simulink model "SF014A_InertiaCmpVel"  (R2013b)
settings: Solver=FixedStepDiscrete  SolverMode=SingleTasking  StartTime=0.0  StopTime=10  FixedStep=0.002  RelTol=1e-3
undefined symbols (not defined in the file): ARCHGLBPRM_2MILLISEC_SEC_F32, ARCHGLBPRM_2PI_ULS_F32, ARCHGLBPRM_PIOVER180_ULS_F32, FLTINJ_INERTIACMPVEL_INERTIACMPCMD, InertiaCmpVelDampgDecelGain, InertiaCmpVelDampgDecelGainFallSlew, InertiaCmpVelDampgGainOffThd, InertiaCmpVelDampgGainOnThd, InertiaCmpVelDecelGainEnaCal, InertiaCmpVelMotInertia, InertiaCmpVelNotchFilStruct, NOTCHFILZEROTHD_ULS_F32, SysGlbPrmSysKineRat, SysGlbPrmTorsBarStfn
libraries: FixdToFloat x13, LnrIntrpn x13, FloatToFixd x9, NxtrAbslt x4, NxtrMath x4, NxtrLim x4, simulink x2, Fil x2
(part 2 of 3)

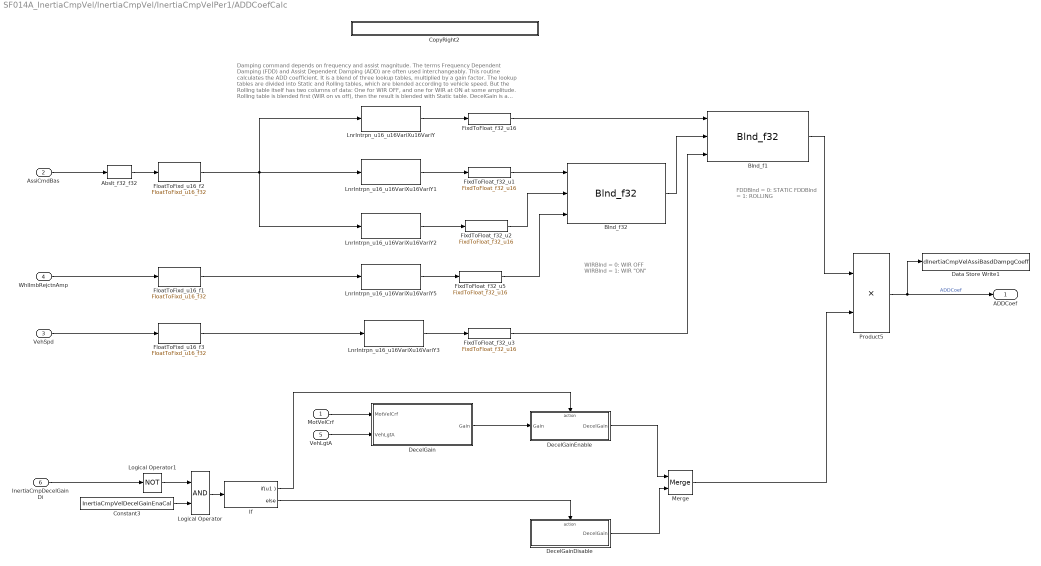
== system SF014A_InertiaCmpVel/InertiaCmpVel/InertiaCmpVelPer1/ADDCoefCalc ==
  note: Damping command depends on frequency and assist magnitude.  The terms Frequency Dependent Damping (FDD) and Assist Dependent Damping (ADD) are
      | often used interchangeably.  This routine calculates the ADD coefficient.  It is a blend of three lookup tables, multiplied by a gain factor.  The lookup tables
      | are divided into Static and Rolling tables, which are blended according to vehicle speed.  But the Rolling table itself has two columns of data:  One for
      | WIR OFF, and one for WIR at ON at some amplitude.  Rolling table is blended first (WIR on vs off), then the result is blended with Static table.
      |
      | DecelGain is a gain applied to damping coefficient when vehicle is aggressively decelerating.
  note: FDDBlnd = 0:  STATIC
      | FDDBlnd = 1:  ROLLING
  note: WIRBlnd = 0:  WIR OFF
      | WIRBlnd = 1:  WIR "ON"
  MotVelCrf : Inport  RequirementInfo="{'linktype_rmi_doors' '0000a52e (/E-STEER Core/SubSystem Specifications/Application Functions/SF014A Inertia Compensation)' '#SF014A_76' 'true' 'REQ:  SF014A_76' '' } %GIDa_dfa7856d_1c61_4589_b30e_750f1eb1645f"
  AssiCmdBas : Inport  RequirementInfo="{'linktype_rmi_doors' '0000a52e (/E-STEER Core/SubSystem Specifications/Application Functions/SF014A Inertia Compensation)' '#SF014A_78' 'true' 'REQ:  SF014A_78' '' } %GIDa_f4af5cbb_f21a_47bc_a42f_a4172f088ae5"  Port=2
  VehSpd : Inport  RequirementInfo="{'linktype_rmi_doors' '0000a52e (/E-STEER Core/SubSystem Specifications/Application Functions/SF014A Inertia Compensation)' '#SF014A_79' 'true' 'REQ:  SF014A_79' '' } %GIDa_a01f0a88_c757_4666_8b69_1ba2342a6170"  Port=3
  WhlImbRejctnAmp : Inport  RequirementInfo="{'linktype_rmi_doors' '0000a52e (/E-STEER Core/SubSystem Specifications/Application Functions/SF014A Inertia Compensation)' '#SF014A_75' 'true' 'REQ:  SF014A_75' '' } %GIDa_85975baa_77aa_432b_910d_ccf6f040e7b8"  Port=4
  VehLgtA : Inport  RequirementInfo="{'linktype_rmi_doors' '0000a52e (/E-STEER Core/SubSystem Specifications/Application Functions/SF014A Inertia Compensation)' '#SF014A_76' 'true' 'REQ:  SF014A_76' '' } %GIDa_8e8fb2ce_6071_474e_9d78_82a4e9de4257"  Port=5
  InertiaCmpDecelGainDi : Inport  RequirementInfo="{'linktype_rmi_doors' '0000a52e (/E-STEER Core/SubSystem Specifications/Application Functions/SF014A Inertia Compensation)' '#SF014A_80' 'true' 'REQ:  SF014A_80' '' } %GIDa_37223524_d1af_4ae4_9408_3e29b9ebc95d"  Port=6
  Abslt_f32_f32 : NxtrAbslt/Abslt_f32_f32  RequirementInfo="{'linktype_rmi_doors' '0000a52e (/E-STEER Core/SubSystem Specifications/Application Functions/SF014A Inertia Compensation)' '#SF014A_78' 'true' 'REQ:  SF014A_78' '' } %GIDa_af49941a_3ea7_4a2b_9c86_73a97f0de25e"  SFunctionSpec=single y1 = Abslt_f32_f32(single u1)
      settings: AttributesFormatString=%<Name>
  Blnd_f1 : NxtrMath/Blnd_f32  RequirementInfo="{'linktype_rmi_doors' '0000a52e (/E-STEER Core/SubSystem Specifications/Application Functions/SF014A Inertia Compensation)' '#SF014A_77' 'true' 'REQ:  SF014A_77' '' } %GIDa_d5de407a_03b4_47a0_a0b7_c554db3a096e"  SFunctionSpec=single y1 = Blnd_f32(single u1, single u2, single u3)  Parameter3=on
      settings: AttributesFormatString=%<Name>
  Blnd_f32 : NxtrMath/Blnd_f32  RequirementInfo="{'linktype_rmi_doors' '0000a52e (/E-STEER Core/SubSystem Specifications/Application Functions/SF014A Inertia Compensation)' '#SF014A_78' 'true' 'REQ:  SF014A_78' '' } %GIDa_356698f6_9f19_4ce5_b1f0_7f4a0c72e2f1"  SFunctionSpec=single y1 = Blnd_f32(single u1, single u2, single u3)  Parameter3=on
      settings: AttributesFormatString=%<Name>
  Constant3 : Constant  RequirementInfo="{'linktype_rmi_doors' '0000a52e (/E-STEER Core/SubSystem Specifications/Application Functions/SF014A Inertia Compensation)' '#SF014A_80' 'true' 'REQ:  SF014A_80' '' } %GIDa_3db1bff2_4e73_4e4e_8f98_1cb123555da8"  Value=InertiaCmpVelDecelGainEnaCal  OutDataTypeStr=boolean
  CopyRight2 : Subsystem  Description=|  mask(Copyright Information){none=on}
      | Copyright info block.                                               
      |                                                                     
      | Place copyright information at the top of every subsystem in design.
      mask prompts: none "No parameters"
      mask help: Place copyright information at the top of every subsystem in design.
      mask Display:
      | NxtrConf = 'Nexteer Confidential';
      | 
      | sys = bdroot; %handle for the current model ("system")
      | first = get_param(sys,'Created');
      | first = first(end-3:end);  %year is last four digits
      | 
      | last = get_param(sys,'LastModifiedDate');
      | if isempty(last)
      |     last = datestr(now,'yyyy');
      | else
      |     last = last(end-3:end);
      | end
      | 
      | if strcmp(first,last)
      |     fprintf('%s -- Copyright %s Nexteer',NxtrConf,first)
      | else
      |     fprintf('%s -- %s%s- %s Nexteer',NxtrConf,char(169),first,last)
      | end
  Data Store Write1 : DataStoreWrite  RequirementInfo="{'linktype_rmi_doors' '0000a52e (/E-STEER Core/SubSystem Specifications/Application Functions/SF014A Inertia Compensation)' '#SF014A_60' 'true' 'REQ:  SF014A_60' '' } %GIDa_70e6b0ec_6545_4ee6_978e_0c2c9530ad6e"  DataStoreName=dInertiaCmpVelAssiBasdDampgCoeff
  DecelGain : Subsystem  RequirementInfo="{'linktype_rmi_doors' '0000a52e (/E-STEER Core/SubSystem Specifications/Application Functions/SF014A Inertia Compensation)' '#SF014A_76' 'true' 'REQ:  SF014A_76' '' } %GIDa_fe0741f4_7d15_4f25_a644_7e9186648f35"
  DecelGainDisable : Subsystem  RequirementInfo="{'linktype_rmi_doors' '0000a52e (/E-STEER Core/SubSystem Specifications/Application Functions/SF014A Inertia Compensation)' '#SF014A_80' 'true' 'REQ:  SF014A_80' '' } %GIDa_c6f53ddd_25da_4339_8f12_9028726cb779"  TreatAsAtomicUnit=on
  DecelGainEnable : Subsystem  RequirementInfo="{'linktype_rmi_doors' '0000a52e (/E-STEER Core/SubSystem Specifications/Application Functions/SF014A Inertia Compensation)' '#SF014A_76' 'true' 'REQ:  SF014A_76' '' } %GIDa_e8d06ef6_defe_46f5_9046_6e95b5ce97d1"  TreatAsAtomicUnit=on
  FixdToFloat_f32_u1 : FixdToFloat/FixdToFloat_f32_u16  RequirementInfo="{'linktype_rmi_doors' '0000a52e (/E-STEER Core/SubSystem Specifications/Application Functions/SF014A Inertia Compensation)' '#SF014A_78' 'true' 'REQ:  SF014A_78' '' } %GIDa_be224bf3_1cd8_491e_b2d0_ce3df0214372"  Param1=16
  FixdToFloat_f32_u16 : FixdToFloat/FixdToFloat_f32_u16  RequirementInfo="{'linktype_rmi_doors' '0000a52e (/E-STEER Core/SubSystem Specifications/Application Functions/SF014A Inertia Compensation)' '#SF014A_77' 'true' 'REQ:  SF014A_77' '' } %GIDa_c4e94e59_b1c9_4f1f_9b7c_e38f7fa17322"  Param1=16
  FixdToFloat_f32_u2 : FixdToFloat/FixdToFloat_f32_u16  RequirementInfo="{'linktype_rmi_doors' '0000a52e (/E-STEER Core/SubSystem Specifications/Application Functions/SF014A Inertia Compensation)' '#SF014A_78' 'true' 'REQ:  SF014A_78' '' } %GIDa_4a949351_78f0_49de_9203_28cc4f0a5888"  Param1=16
  FixdToFloat_f32_u3 : FixdToFloat/FixdToFloat_f32_u16  RequirementInfo="{'linktype_rmi_doors' '0000a52e (/E-STEER Core/SubSystem Specifications/Application Functions/SF014A Inertia Compensation)' '#SF014A_79' 'true' 'REQ:  SF014A_79' '' } %GIDa_c7f288c6_8432_4513_b88a_c2722fb22052"  Param1=15
  FixdToFloat_f32_u5 : FixdToFloat/FixdToFloat_f32_u16  RequirementInfo="{'linktype_rmi_doors' '0000a52e (/E-STEER Core/SubSystem Specifications/Application Functions/SF014A Inertia Compensation)' '#SF014A_75' 'true' 'REQ:  SF014A_75' '' } %GIDa_6d830592_a8f2_4eeb_a9c7_97a648ca295c"  Param1=15
  FloatToFixd_u16_f1 : FloatToFixd/FloatToFixd_u16_f32  RequirementInfo="{'linktype_rmi_doors' '0000a52e (/E-STEER Core/SubSystem Specifications/Application Functions/SF014A Inertia Compensation)' '#SF014A_75' 'true' 'REQ:  SF014A_75' '' } %GIDa_fb611f55_8f4e_4c3e_a41a_8829889732ad"  Param1=12
  FloatToFixd_u16_f2 : FloatToFixd/FloatToFixd_u16_f32  RequirementInfo="{'linktype_rmi_doors' '0000a52e (/E-STEER Core/SubSystem Specifications/Application Functions/SF014A Inertia Compensation)' '#SF014A_78' 'true' 'REQ:  SF014A_78' '' } %GIDa_6e220007_6fc8_492c_98e2_22994a0581f2"  Param1=12
  FloatToFixd_u16_f3 : FloatToFixd/FloatToFixd_u16_f32  RequirementInfo="{'linktype_rmi_doors' '0000a52e (/E-STEER Core/SubSystem Specifications/Application Functions/SF014A Inertia Compensation)' '#SF014A_79' 'true' 'REQ:  SF014A_79' '' } %GIDa_9965882c_9557_4904_863f_c266d2ac13fd"  Param1=7
  If : If  RequirementInfo="{'linktype_rmi_doors' '0000a52e (/E-STEER Core/SubSystem Specifications/Application Functions/SF014A Inertia Compensation)' '#SF014A_80' 'true' 'REQ:  SF014A_80' '' } %GIDa_47807508_1654_41c2_b488_a483d15670e6"  IfExpression=u1
  LnrIntrpn_u16_u16VariXu16VariY : LnrIntrpn/LnrIntrpn_u16_u16VariXu16VariY  RequirementInfo="{'linktype_rmi_doors' '0000a52e (/E-STEER Core/SubSystem Specifications/Application Functions/SF014A Inertia Compensation)' '#SF014A_77' 'true' 'REQ:  SF014A_77' '' } %GIDa_6ef6b099_ff5f_4012_a091_ab948f1fc6d8"  XTbl=InertiaCmpVelAssiBasdDampgCoeffX  YTbl=InertiaCmpVelAssiBasdDampgStatY
      settings: AttributesFormatString=Lnr ( u16VariX , u16VariY )
  LnrIntrpn_u16_u16VariXu16VariY1 : LnrIntrpn/LnrIntrpn_u16_u16VariXu16VariY  RequirementInfo="{'linktype_rmi_doors' '0000a52e (/E-STEER Core/SubSystem Specifications/Application Functions/SF014A Inertia Compensation)' '#SF014A_78' 'true' 'REQ:  SF014A_78' '' } %GIDa_c5c7e8fc_1b3e_4605_b3a0_1b80b5584e05"  XTbl=InertiaCmpVelAssiBasdDampgCoeffX  YTbl=InertiaCmpVelAssiBasdDampgRollgY
      settings: AttributesFormatString=Lnr ( u16VariX , u16VariY )
  LnrIntrpn_u16_u16VariXu16VariY2 : LnrIntrpn/LnrIntrpn_u16_u16VariXu16VariY  RequirementInfo="{'linktype_rmi_doors' '0000a52e (/E-STEER Core/SubSystem Specifications/Application Functions/SF014A Inertia Compensation)' '#SF014A_78' 'true' 'REQ:  SF014A_78' '' } %GIDa_0a7a390e_dded_4f14_85ed_d87f43b0e08a"  XTbl=InertiaCmpVelAssiBasdDampgCoeffX  YTbl=InertiaCmpVelAssiBasdDampgRollgWhlImbRejctnOnY
      settings: AttributesFormatString=Lnr ( u16VariX , u16VariY )
  LnrIntrpn_u16_u16VariXu16VariY3 : LnrIntrpn/LnrIntrpn_u16_u16VariXu16VariY  RequirementInfo="{'linktype_rmi_doors' '0000a52e (/E-STEER Core/SubSystem Specifications/Application Functions/SF014A Inertia Compensation)' '#SF014A_79' 'true' 'REQ:  SF014A_79' '' } %GIDa_3f6ebfaf_e532_492e_a591_116aa8f65af2"  XTbl=SysGlbPrmVehSpdBilnrSeln  YTbl=InertiaCmpVelDampgSpdBlndY
      settings: AttributesFormatString=Lnr ( u16VariX , u16VariY )
  LnrIntrpn_u16_u16VariXu16VariY5 : LnrIntrpn/LnrIntrpn_u16_u16VariXu16VariY  RequirementInfo="{'linktype_rmi_doors' '0000a52e (/E-STEER Core/SubSystem Specifications/Application Functions/SF014A Inertia Compensation)' '#SF014A_75' 'true' 'REQ:  SF014A_75' '' } %GIDa_bf9922ec_f3a9_44c1_9df9_2bc58a5a9adc"  XTbl=InertiaCmpVelDampgWhlImbRejctnBlndX  YTbl=InertiaCmpVelDampgWhlImbRejctnBlndY
      settings: AttributesFormatString=Lnr ( u16VariX , u16VariY )
  Logical Operator : Logic  RequirementInfo="{'linktype_rmi_doors' '0000a52e (/E-STEER Core/SubSystem Specifications/Application Functions/SF014A Inertia Compensation)' '#SF014A_80' 'true' 'REQ:  SF014A_80' '' } %GIDa_3d748ccb_4553_46fa_830c_9d4437689221"  AllPortsSameDT=off  OutDataTypeStr=boolean
  Logical Operator1 : Logic  RequirementInfo="{'linktype_rmi_doors' '0000a52e (/E-STEER Core/SubSystem Specifications/Application Functions/SF014A Inertia Compensation)' '#SF014A_80' 'true' 'REQ:  SF014A_80' '' } %GIDa_bef89e48_fbb8_4e23_aa0f_f13752227eac"  Operator=NOT  AllPortsSameDT=off  OutDataTypeStr=boolean
  Merge : Merge
  Product5 : Product  RequirementInfo="{'linktype_rmi_doors' '0000a52e (/E-STEER Core/SubSystem Specifications/Application Functions/SF014A Inertia Compensation)' '#SF014A_60' 'true' 'REQ:  SF014A_60' '' } %GIDa_a9a1c5c6_e001_4095_82f0_6dff06eebe1a"  SaturateOnIntegerOverflow=on  OutDataTypeStr=Inherit: Same as first input
  ADDCoef : Outport  RequirementInfo="{'linktype_rmi_doors' '0000a52e (/E-STEER Core/SubSystem Specifications/Application Functions/SF014A Inertia Compensation)' '#SF014A_60' 'true' 'REQ:  SF014A_60' '' } %GIDa_baacfa22_4b61_476c_9be4_d90fd9ee3dcb"
  wires:
  AssiCmdBas/1 -> Abslt_f32_f32/1
  Product5/1 -> Data Store Write1/1, ADDCoef/1  "ADDCoef"
  MotVelCrf/1 -> DecelGain/1(MotVelCrf)
  VehSpd/1 -> FloatToFixd_u16_f3/1
  WhlImbRejctnAmp/1 -> FloatToFixd_u16_f1/1
  Abslt_f32_f32/1 -> FloatToFixd_u16_f2/1
  VehLgtA/1 -> DecelGain/2(VehLgtA)
  LnrIntrpn_u16_u16VariXu16VariY/1 -> FixdToFloat_f32_u16/1
  LnrIntrpn_u16_u16VariXu16VariY1/1 -> FixdToFloat_f32_u1/1
  LnrIntrpn_u16_u16VariXu16VariY2/1 -> FixdToFloat_f32_u2/1
  FloatToFixd_u16_f2/1 -> LnrIntrpn_u16_u16VariXu16VariY2/1, LnrIntrpn_u16_u16VariXu16VariY/1, LnrIntrpn_u16_u16VariXu16VariY1/1
  FixdToFloat_f32_u1/1 -> Blnd_f32/1
  FixdToFloat_f32_u2/1 -> Blnd_f32/2
  LnrIntrpn_u16_u16VariXu16VariY5/1 -> FixdToFloat_f32_u5/1
  FloatToFixd_u16_f1/1 -> LnrIntrpn_u16_u16VariXu16VariY5/1
  FixdToFloat_f32_u5/1 -> Blnd_f32/3
  Blnd_f1/1 -> Product5/1
  LnrIntrpn_u16_u16VariXu16VariY3/1 -> FixdToFloat_f32_u3/1
  FloatToFixd_u16_f3/1 -> LnrIntrpn_u16_u16VariXu16VariY3/1
  FixdToFloat_f32_u16/1 -> Blnd_f1/1
  Blnd_f32/1 -> Blnd_f1/2
  FixdToFloat_f32_u3/1 -> Blnd_f1/3
  DecelGain/1(Gain) -> DecelGainEnable/1(Gain)
  InertiaCmpDecelGainDi/1 -> Logical Operator1/1
  Merge/1 -> Product5/2
  DecelGainDisable/1(DecelGain) -> Merge/2
  DecelGainEnable/1(DecelGain) -> Merge/1
  If/1 -> DecelGainEnable/Action
  If/2 -> DecelGainDisable/Action
  Constant3/1 -> Logical Operator/2
  Logical Operator1/1 -> Logical Operator/1
  Logical Operator/1 -> If/1

== system SF014A_InertiaCmpVel/InertiaCmpVel/InertiaCmpVelPer1/CopyRight2 ==

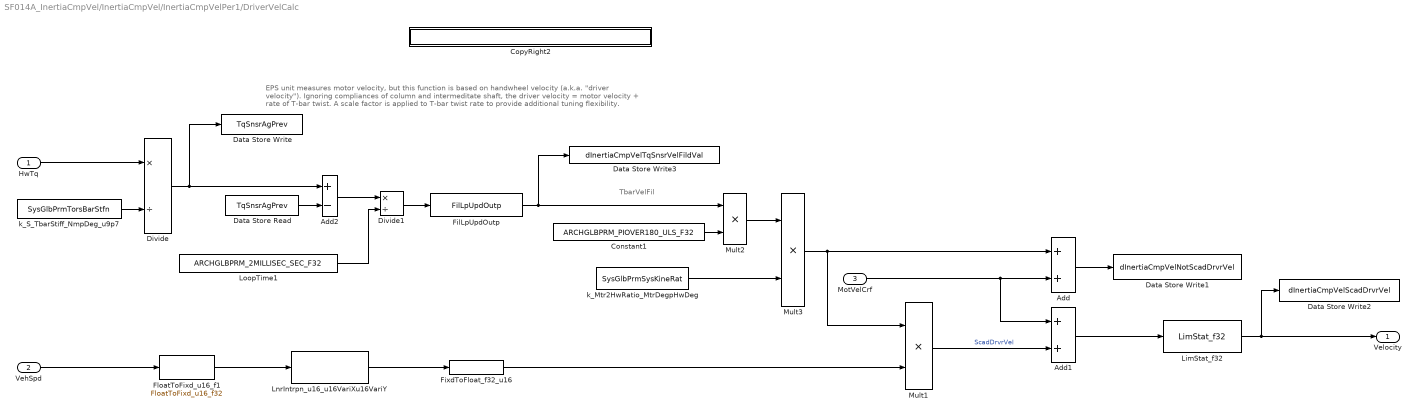
== system SF014A_InertiaCmpVel/InertiaCmpVel/InertiaCmpVelPer1/DriverVelCalc ==
  note: TbarVelFil
  note: EPS unit measures motor velocity, but this function is based on handwheel velocity (a.k.a. "driver velocity").  Ignoring compliances of column and intermeditate shaft, the
      | driver velocity = motor velocity + rate of T-bar twist.  A scale factor is applied to T-bar twist rate to provide additional tuning flexibility.
  HwTq : Inport  RequirementInfo="{'linktype_rmi_doors' '0000a52e (/E-STEER Core/SubSystem Specifications/Application Functions/SF014A Inertia Compensation)' '#SF014A_70' 'true' 'REQ:  SF014A_70' '' } %GIDa_ac2c02ba_8ee6_417c_b9af_1a2925850df1"
  VehSpd : Inport  RequirementInfo="{'linktype_rmi_doors' '0000a52e (/E-STEER Core/SubSystem Specifications/Application Functions/SF014A Inertia Compensation)' '#SF014A_73' 'true' 'REQ:  SF014A_73' '' } %GIDa_5ab90069_7b23_42c3_b4f4_f069992e6f81"  Port=2
  MotVelCrf : Inport  RequirementInfo="{'linktype_rmi_doors' '0000a52e (/E-STEER Core/SubSystem Specifications/Application Functions/SF014A Inertia Compensation)' '#SF014A_72' 'true' 'REQ:  SF014A_72' '' } %GIDa_c3842865_6d96_477b_a623_1016ce55a84b"  Port=3
  Add : Sum  RequirementInfo={} %GIDa_6dd307c5_b434_4b5e_9d26_e92cac49f28a
  Add1 : Sum  RequirementInfo="{'linktype_rmi_doors' '0000a52e (/E-STEER Core/SubSystem Specifications/Application Functions/SF014A Inertia Compensation)' '#SF014A_72' 'true' 'REQ:  SF014A_72' '' } %GIDa_04e893ef_79c8_4adc_8c1f_0d7246edb46a"
  Add2 : Sum  RequirementInfo="{'linktype_rmi_doors' '0000a52e (/E-STEER Core/SubSystem Specifications/Application Functions/SF014A Inertia Compensation)' '#SF014A_70' 'true' 'REQ:  SF014A_70' '' } %GIDa_b3518012_7564_4a99_a0ea_cf2ec37a4818"  Inputs=+-
  Constant1 : Constant  RequirementInfo="{'linktype_rmi_doors' '0000a52e (/E-STEER Core/SubSystem Specifications/Application Functions/SF014A Inertia Compensation)' '#SF014A_70' 'true' 'REQ:  SF014A_70' '' } %GIDa_8d7cf654_9361_4608_a7ae_b88b718702a6"  Value=ARCHGLBPRM_PIOVER180_ULS_F32
  CopyRight2 : Subsystem  Description=|  mask(Copyright Information){none=on}
      | Copyright info block.                                               
      |                                                                     
      | Place copyright information at the top of every subsystem in design.
      mask prompts: none "No parameters"
      mask help: Place copyright information at the top of every subsystem in design.
      mask Display:
      | NxtrConf = 'Nexteer Confidential';
      | 
      | sys = bdroot; %handle for the current model ("system")
      | first = get_param(sys,'Created');
      | first = first(end-3:end);  %year is last four digits
      | 
      | last = get_param(sys,'LastModifiedDate');
      | if isempty(last)
      |     last = datestr(now,'yyyy');
      | else
      |     last = last(end-3:end);
      | end
      | 
      | if strcmp(first,last)
      |     fprintf('%s -- Copyright %s Nexteer',NxtrConf,first)
      | else
      |     fprintf('%s -- %s%s- %s Nexteer',NxtrConf,char(169),first,last)
      | end
  Data Store Read : DataStoreRead  RequirementInfo="{'linktype_rmi_doors' '0000a52e (/E-STEER Core/SubSystem Specifications/Application Functions/SF014A Inertia Compensation)' '#SF014A_70' 'true' 'REQ:  SF014A_70' '' } %GIDa_36e69ac2_9dd5_46cf_a9c8_b935e242cb27"  Priority=1  DataStoreName=TqSnsrAgPrev
      settings: AttributesFormatString=Priority%<priority>
  Data Store Write : DataStoreWrite  RequirementInfo="{'linktype_rmi_doors' '0000a52e (/E-STEER Core/SubSystem Specifications/Application Functions/SF014A Inertia Compensation)' '#SF014A_70' 'true' 'REQ:  SF014A_70' '' } %GIDa_82ecf4fd_4e6c_4fd4_9da5_4862ee27ce65"  Priority=2  DataStoreName=TqSnsrAgPrev
      settings: AttributesFormatString=priority %<Priority>
  Data Store Write1 : DataStoreWrite  RequirementInfo={} %GIDa_bfd9e8d0_f312_434d_a5ad_bac24325db40  DataStoreName=dInertiaCmpVelNotScadDrvrVel
  Data Store Write2 : DataStoreWrite  DataStoreName=dInertiaCmpVelScadDrvrVel
  Data Store Write3 : DataStoreWrite  RequirementInfo="{'linktype_rmi_doors' '0000a52e (/E-STEER Core/SubSystem Specifications/Application Functions/SF014A Inertia Compensation)' '#SF014A_70' 'true' 'REQ:  SF014A_70' '' } %GIDa_aafe90dd_974e_4ff5_9a1d_a2e136272378"  DataStoreName=dInertiaCmpVelTqSnsrVelFildVal
  Divide : Product  RequirementInfo="{'linktype_rmi_doors' '0000a52e (/E-STEER Core/SubSystem Specifications/Application Functions/SF014A Inertia Compensation)' '#SF014A_70' 'true' 'REQ:  SF014A_70' '' } %GIDa_158430a0_bd87_4716_93c4_82a6a6e927b1"  Inputs=*/
  Divide1 : Product  RequirementInfo="{'linktype_rmi_doors' '0000a52e (/E-STEER Core/SubSystem Specifications/Application Functions/SF014A Inertia Compensation)' '#SF014A_70' 'true' 'REQ:  SF014A_70' '' } %GIDa_6eb80e6c_ab3f_408d_9a71_5d2d41187984"  Inputs=*/
  FilLpUpdOutp : Fil/FilLpUpdOutp  RequirementInfo="{'linktype_rmi_doors' '0000a52e (/E-STEER Core/SubSystem Specifications/Application Functions/SF014A Inertia Compensation)' '#SF014A_70' 'true' 'REQ:  SF014A_70' '' } %GIDa_58f1a0c2_f235_4076_92f9_f89e3f545d25"  StVar=TqSnsrVelFil
      settings: AttributesFormatString=StVar: %<StVar>
  FixdToFloat_f32_u16 : FixdToFloat/FixdToFloat_f32_u16  RequirementInfo="{'linktype_rmi_doors' '0000a52e (/E-STEER Core/SubSystem Specifications/Application Functions/SF014A Inertia Compensation)' '#SF014A_73' 'true' 'REQ:  SF014A_73' '' } %GIDa_999c9d2b_355a_4301_82f1_ecfecb6502c1"  Param1=14
  FloatToFixd_u16_f1 : FloatToFixd/FloatToFixd_u16_f32  RequirementInfo="{'linktype_rmi_doors' '0000a52e (/E-STEER Core/SubSystem Specifications/Application Functions/SF014A Inertia Compensation)' '#SF014A_73' 'true' 'REQ:  SF014A_73' '' } %GIDa_6923e43e_2e8b_4d16_953d_56e5e4b8b0af"  Param1=7
  LimStat_f32 : NxtrLim/LimStat_f32  RequirementInfo="{'linktype_rmi_doors' '0000a52e (/E-STEER Core/SubSystem Specifications/Application Functions/SF014A Inertia Compensation)' '#SF014A_71' 'true' 'REQ:  SF014A_71' '' } %GIDa_c63e7996_e378_4888_9cc5_19a0c9093416"  LoLim=MOTVELLOLIM_MOTRADPERSEC_F32  HiLim=MOTVELHILIM_MOTRADPERSEC_F32
      settings: AttributesFormatString=|
      | Low Limit: %<LoLim>
      | High Limit:%<HiLim>
  LnrIntrpn_u16_u16VariXu16VariY : LnrIntrpn/LnrIntrpn_u16_u16VariXu16VariY  RequirementInfo="{'linktype_rmi_doors' '0000a52e (/E-STEER Core/SubSystem Specifications/Application Functions/SF014A Inertia Compensation)' '#SF014A_73' 'true' 'REQ:  SF014A_73' '' } %GIDa_ada56006_9441_4287_84b1_d0c49486caba"  XTbl=SysGlbPrmVehSpdBilnrSeln  YTbl=InertiaCmpVelTqSnsrVelSca
      settings: AttributesFormatString=Lnr ( u16VariX , u16VariY )
  LoopTime1 : Constant  RequirementInfo="{'linktype_rmi_doors' '0000a52e (/E-STEER Core/SubSystem Specifications/Application Functions/SF014A Inertia Compensation)' '#SF014A_70' 'true' 'REQ:  SF014A_70' '' } %GIDa_f4414744_eff0_447c_b77a_b1837c25c653"  Value=ARCHGLBPRM_2MILLISEC_SEC_F32
  Mult1 : Product  RequirementInfo="{'linktype_rmi_doors' '0000a52e (/E-STEER Core/SubSystem Specifications/Application Functions/SF014A Inertia Compensation)' '#SF014A_73' 'true' 'REQ:  SF014A_73' '' } %GIDa_5cc158a1_2d3a_466c_9940_b9d9a843b400"  Inputs=**
  Mult2 : Product  RequirementInfo="{'linktype_rmi_doors' '0000a52e (/E-STEER Core/SubSystem Specifications/Application Functions/SF014A Inertia Compensation)' '#SF014A_70' 'true' 'REQ:  SF014A_70' '' } %GIDa_246acc40_e3a1_465e_aad8_8c68179e5a7d"  Inputs=**
  Mult3 : Product  RequirementInfo="{'linktype_rmi_doors' '0000a52e (/E-STEER Core/SubSystem Specifications/Application Functions/SF014A Inertia Compensation)' '#SF014A_70' 'true' 'REQ:  SF014A_70' '' } %GIDa_d2f3bae5_f43f_4edc_a03c_8c9115f5dd9a"  Inputs=**
  k_Mtr2HwRatio_MtrDegpHwDeg : Constant  RequirementInfo="{'linktype_rmi_doors' '0000a52e (/E-STEER Core/SubSystem Specifications/Application Functions/SF014A Inertia Compensation)' '#SF014A_70' 'true' 'REQ:  SF014A_70' '' } %GIDa_b6e50b20_b12a_4321_9dac_8363b00120b2"  Value=SysGlbPrmSysKineRat
  k_S_TbarStiff_NmpDeg_u9p7 : Constant  RequirementInfo="{'linktype_rmi_doors' '0000a52e (/E-STEER Core/SubSystem Specifications/Application Functions/SF014A Inertia Compensation)' '#SF014A_70' 'true' 'REQ:  SF014A_70' '' } %GIDa_2fa8f7f8_e6c0_4ab0_b79b_0aeb2cdc1d20"  Value=SysGlbPrmTorsBarStfn
  Velocity : Outport
  wires:
  HwTq/1 -> Divide/1
  k_S_TbarStiff_NmpDeg_u9p7/1 -> Divide/2
  Divide/1 -> Add2/1, Data Store Write/1
  Divide1/1 -> FilLpUpdOutp/1
  Mult2/1 -> Mult3/1
  k_Mtr2HwRatio_MtrDegpHwDeg/1 -> Mult3/2
  Mult3/1 -> Mult1/1, Add/1
  Add/1 -> Data Store Write1/1
  LnrIntrpn_u16_u16VariXu16VariY/1 -> FixdToFloat_f32_u16/1
  FilLpUpdOutp/1 -> Data Store Write3/1, Mult2/1
  Add2/1 -> Divide1/1
  LoopTime1/1 -> Divide1/2
  Mult1/1 -> Add1/2  "ScadDrvrVel"
  VehSpd/1 -> FloatToFixd_u16_f1/1
  MotVelCrf/1 -> Add1/1, Add/2
  Data Store Read/1 -> Add2/2
  FloatToFixd_u16_f1/1 -> LnrIntrpn_u16_u16VariXu16VariY/1
  FixdToFloat_f32_u16/1 -> Mult1/2
  Constant1/1 -> Mult2/2
  LimStat_f32/1 -> Velocity/1, Data Store Write2/1
  Add1/1 -> LimStat_f32/1

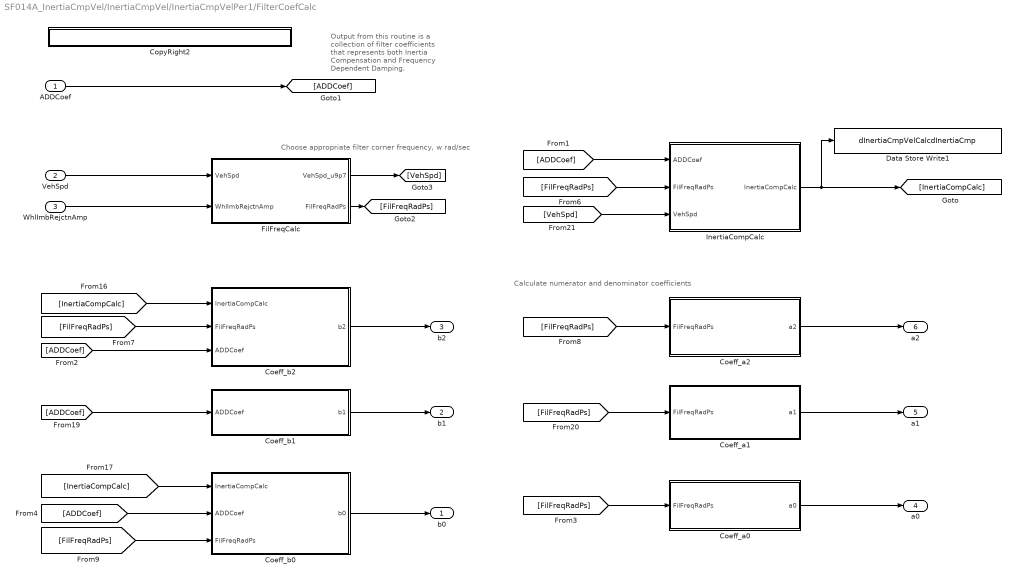
== system SF014A_InertiaCmpVel/InertiaCmpVel/InertiaCmpVelPer1/FilterCoefCalc ==
  note: Choose appropriate filter corner frequency, w rad/sec
  note: Calculate numerator and denominator coefficients
  note: Output from this routine is a collection of filter coefficients that represents both Inertia Compensation and Frequency Dependent Damping.
  ADDCoef : Inport
  VehSpd : Inport  Port=2
  WhlImbRejctnAmp : Inport  Port=3
  Coeff_a0 : Subsystem
  Coeff_a1 : Subsystem
  Coeff_a2 : Subsystem
  Coeff_b0 : Subsystem
  Coeff_b1 : Subsystem
  Coeff_b2 : Subsystem
  CopyRight2 : Subsystem  Description=|  mask(Copyright Information){none=on}
      | Copyright info block.                                               
      |                                                                     
      | Place copyright information at the top of every subsystem in design.
      mask prompts: none "No parameters"
      mask help: Place copyright information at the top of every subsystem in design.
      mask Display:
      | NxtrConf = 'Nexteer Confidential';
      | 
      | sys = bdroot; %handle for the current model ("system")
      | first = get_param(sys,'Created');
      | first = first(end-3:end);  %year is last four digits
      | 
      | last = get_param(sys,'LastModifiedDate');
      | if isempty(last)
      |     last = datestr(now,'yyyy');
      | else
      |     last = last(end-3:end);
      | end
      | 
      | if strcmp(first,last)
      |     fprintf('%s -- Copyright %s Nexteer',NxtrConf,first)
      | else
      |     fprintf('%s -- %s%s- %s Nexteer',NxtrConf,char(169),first,last)
      | end
  Data Store Write1 : DataStoreWrite  DataStoreName=dInertiaCmpVelCalcdInertiaCmp
  FilFreqCalc : Subsystem
  InertiaCompCalc : Subsystem
  b0 : Outport
  b1 : Outport  Port=2
  b2 : Outport  Port=3
  a0 : Outport  Port=4
  a1 : Outport  Port=5
  a2 : Outport  Port=6
  wires:
  ADDCoef/1 -> [ADDCoef]
  [FilFreqRadPs] -> Coeff_a2/1(FilFreqRadPs)
  Coeff_a2/1(a2) -> a2/1
  [FilFreqRadPs] -> Coeff_a1/1(FilFreqRadPs)
  Coeff_a1/1(a1) -> a1/1
  [ADDCoef] -> Coeff_b1/1(ADDCoef)
  Coeff_b1/1(b1) -> b1/1
  [InertiaCompCalc] -> Coeff_b2/1(InertiaCompCalc)
  [ADDCoef] -> Coeff_b2/3(ADDCoef)
  [FilFreqRadPs] -> Coeff_b2/2(" FilFreqRadPs")
  Coeff_b2/1(b2) -> b2/1
  [FilFreqRadPs] -> Coeff_a0/1(FilFreqRadPs)
  Coeff_a0/1(a0) -> a0/1
  [InertiaCompCalc] -> Coeff_b0/1(InertiaCompCalc)
  [ADDCoef] -> Coeff_b0/2(ADDCoef)
  [FilFreqRadPs] -> Coeff_b0/3(FilFreqRadPs)
  Coeff_b0/1(b0) -> b0/1
  InertiaCompCalc/1(InertiaCompCalc) -> Data Store Write1/1, [InertiaCompCalc]
  [ADDCoef] -> InertiaCompCalc/1(ADDCoef)
  [FilFreqRadPs] -> InertiaCompCalc/2(FilFreqRadPs)
  [VehSpd] -> InertiaCompCalc/3(VehSpd)
  VehSpd/1 -> FilFreqCalc/1(VehSpd)
  WhlImbRejctnAmp/1 -> FilFreqCalc/2(WhlImbRejctnAmp)
  FilFreqCalc/2(FilFreqRadPs) -> [FilFreqRadPs]
  FilFreqCalc/1(VehSpd_u9p7) -> [VehSpd]

== system SF014A_InertiaCmpVel/InertiaCmpVel/InertiaCmpVelPer1/FltInj_f32 ==
  note: Inport #2 must be constant
      | Const: FltInjectionLocType
  note: EA4.x Fault Injection
  note: This block requires no modification by FDD author.
      |
      | This block does not actually simulate any fault injection.  It is simply a pass-thru.
      |
      | The Const port (#2) simply terminates its signal, but we are trying to force the FDD author
      | to properly use the FltInjectionLocType enumeration in FDD model.
  Signal : Inport
  Const : Inport  Port=2
  Terminator : Terminator
  Out1 : Outport
  wires:
  Const/1 -> Terminator/1
  Signal/1 -> Out1/1

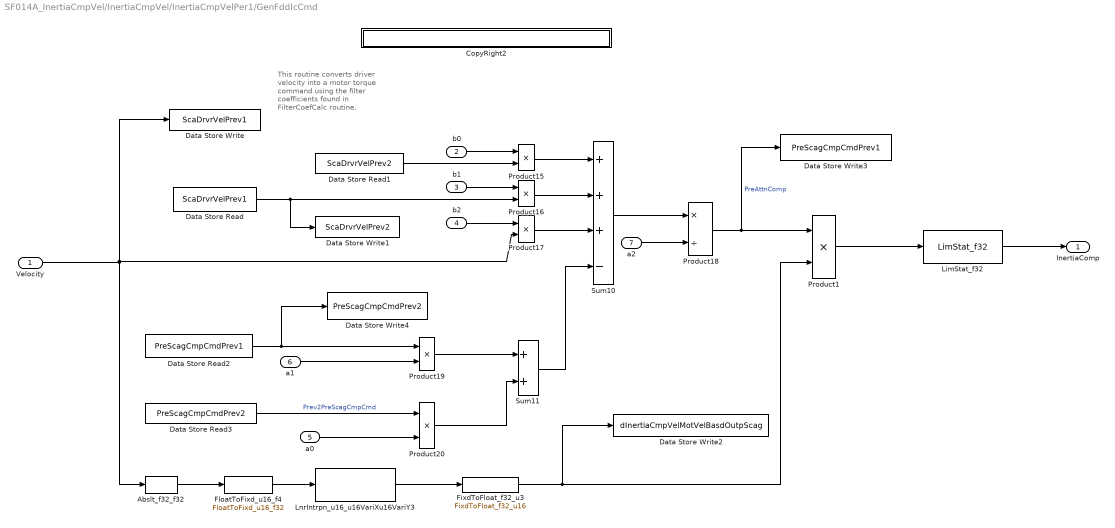
== system SF014A_InertiaCmpVel/InertiaCmpVel/InertiaCmpVelPer1/GenFddIcCmd ==
  note: This routine converts driver velocity into a motor torque command using the filter coefficients found in FilterCoefCalc routine.
  Velocity : Inport
  b0 : Inport  Port=2
  b1 : Inport  Port=3
  b2 : Inport  Port=4
  a0 : Inport  Port=5
  a1 : Inport  Port=6
  a2 : Inport  Port=7
  Abslt_f32_f32 : NxtrAbslt/Abslt_f32_f32  SFunctionSpec=single y1 = Abslt_f32_f32(single u1)
      settings: AttributesFormatString=%<Name>
  CopyRight2 : Subsystem  Description=|  mask(Copyright Information){none=on}
      | Copyright info block.                                               
      |                                                                     
      | Place copyright information at the top of every subsystem in design.
      mask prompts: none "No parameters"
      mask help: Place copyright information at the top of every subsystem in design.
      mask Display:
      | NxtrConf = 'Nexteer Confidential';
      | 
      | sys = bdroot; %handle for the current model ("system")
      | first = get_param(sys,'Created');
      | first = first(end-3:end);  %year is last four digits
      | 
      | last = get_param(sys,'LastModifiedDate');
      | if isempty(last)
      |     last = datestr(now,'yyyy');
      | else
      |     last = last(end-3:end);
      | end
      | 
      | if strcmp(first,last)
      |     fprintf('%s -- Copyright %s Nexteer',NxtrConf,first)
      | else
      |     fprintf('%s -- %s%s- %s Nexteer',NxtrConf,char(169),first,last)
      | end
  Data Store Read : DataStoreRead  DataStoreName=ScaDrvrVelPrev1
      settings: AttributesFormatString=priority 1%<Priority>
  Data Store Read1 : DataStoreRead  DataStoreName=ScaDrvrVelPrev2
      settings: AttributesFormatString=priority 1 %<Priority>
  Data Store Read2 : DataStoreRead  DataStoreName=PreScagCmpCmdPrev1
      settings: AttributesFormatString=priority 1%<Priority>
  Data Store Read3 : DataStoreRead  DataStoreName=PreScagCmpCmdPrev2
      settings: AttributesFormatString=priority 1%<Priority>
  Data Store Write : DataStoreWrite  DataStoreName=ScaDrvrVelPrev1
      settings: AttributesFormatString=priority 2%<Priority>
  Data Store Write1 : DataStoreWrite  DataStoreName=ScaDrvrVelPrev2
      settings: AttributesFormatString=priority 2%<Priority>
  Data Store Write2 : DataStoreWrite  DataStoreName=dInertiaCmpVelMotVelBasdOutpScag
  Data Store Write3 : DataStoreWrite  DataStoreName=PreScagCmpCmdPrev1
      settings: AttributesFormatString=priority 2 %<Priority>
  Data Store Write4 : DataStoreWrite  DataStoreName=PreScagCmpCmdPrev2
      settings: AttributesFormatString=priority 2%<Priority>
  FixdToFloat_f32_u3 : FixdToFloat/FixdToFloat_f32_u16  Param1=15
  FloatToFixd_u16_f4 : FloatToFixd/FloatToFixd_u16_f32  Param1=4
  LimStat_f32 : NxtrLim/LimStat_f32  LoLim=SYSGLBPRM_MOTTQCMDLOLIM_MOTNWTMTR_F32  HiLim=SYSGLBPRM_MOTTQCMDHILIM_MOTNWTMTR_F32
      settings: AttributesFormatString=|
      | Low Limit: %<LoLim>
      | High Limit:%<HiLim>
  LnrIntrpn_u16_u16VariXu16VariY3 : LnrIntrpn/LnrIntrpn_u16_u16VariXu16VariY  XTbl=InertiaCmpVelMotVelBasdOutpScagX  YTbl=InertiaCmpVelMotVelBasdOutpScagY
      settings: AttributesFormatString=Lnr ( u16VariX , u16VariY )
  Product{1,15..17,19..20} (6 alike) : Product  RndMeth=Zero  OutDataTypeStr=Inherit: Same as first input
  Product18 : Product  Inputs=*/  RndMeth=Zero  OutDataTypeStr=Inherit: Same as first input
  Sum10 : Sum  Inputs=+++-  OutDataTypeStr=Inherit: Same as first input
  Sum11 : Sum  OutDataTypeStr=Inherit: Same as first input
  InertiaComp : Outport
  wires:
  Velocity/1 -> Abslt_f32_f32/1, Data Store Write/1, Product17/2
  b0/1 -> Product15/1
  b1/1 -> Product16/1
  b2/1 -> Product17/1
  Product15/1 -> Sum10/1
  Product16/1 -> Sum10/2
  Product17/1 -> Sum10/3
  Sum10/1 -> Product18/1
  a2/1 -> Product18/2
  Product18/1 -> Product1/1, Data Store Write3/1  "PreAttnComp"
  Sum11/1 -> Sum10/4
  a1/1 -> Product19/2
  Data Store Read3/1 -> Product20/1  "Prev2PreScagCmpCmd"
  a0/1 -> Product20/2
  Product19/1 -> Sum11/1
  Product20/1 -> Sum11/2
  FixdToFloat_f32_u3/1 -> Product1/2, Data Store Write2/1
  Product1/1 -> LimStat_f32/1
  Data Store Read/1 -> Product16/2, Data Store Write1/1
  Data Store Read1/1 -> Product15/2
  Data Store Read2/1 -> Product19/1, Data Store Write4/1
  LnrIntrpn_u16_u16VariXu16VariY3/1 -> FixdToFloat_f32_u3/1
  FloatToFixd_u16_f4/1 -> LnrIntrpn_u16_u16VariXu16VariY3/1
  Abslt_f32_f32/1 -> FloatToFixd_u16_f4/1
  LimStat_f32/1 -> InertiaComp/1

== system SF014A_InertiaCmpVel/InertiaCmpVel/InertiaCmpVelPer1/Inertia Comp Notch Compensation ==
  InertiaComp : Inport
  VehSpd : Inport  RequirementInfo="{'linktype_rmi_doors' '0000a52e (/E-STEER Core/SubSystem Specifications/Application Functions/SF014A Inertia Compensation)' '#SF014A_92' 'true' 'REQ:  SF014A_92' '' } %GIDa_e8b6c8ac_b20e_4ac2_915b_a1a028e3b1ff"  Port=2
  Blnd_f32 : NxtrMath/Blnd_f32  RequirementInfo="{'linktype_rmi_doors' '0000a52e (/E-STEER Core/SubSystem Specifications/Application Functions/SF014A Inertia Compensation)' '#SF014A_91' 'true' 'REQ:  SF014A_91' '' } %GIDa_912fc06a_b76c_46f6_8e4f_42a646a5c181"  SFunctionSpec=single y1 = Blnd_f32(single u1, single u2, single u3)  Parameter3=on
      settings: AttributesFormatString=%<Name>
  CopyRight2 : Subsystem  Description=|  mask(Copyright Information){none=on}
      | Copyright info block.                                               
      |                                                                     
      | Place copyright information at the top of every subsystem in design.
      mask prompts: none "No parameters"
      mask help: Place copyright information at the top of every subsystem in design.
      mask Display:
      | NxtrConf = 'Nexteer Confidential';
      | 
      | sys = bdroot; %handle for the current model ("system")
      | first = get_param(sys,'Created');
      | first = first(end-3:end);  %year is last four digits
      | 
      | last = get_param(sys,'LastModifiedDate');
      | if isempty(last)
      |     last = datestr(now,'yyyy');
      | else
      |     last = last(end-3:end);
      | end
      | 
      | if strcmp(first,last)
      |     fprintf('%s -- Copyright %s Nexteer',NxtrConf,first)
      | else
      |     fprintf('%s -- %s%s- %s Nexteer',NxtrConf,char(169),first,last)
      | end
  Data Store Write1 : DataStoreWrite  DataStoreName=dInertiaCmpVelNotchBlndVal
  Data Store Write2 : DataStoreWrite  DataStoreName=dInertiaCmpVelNotchOutpVal
  Data Store Write3 : DataStoreWrite  DataStoreName=dInertiaCmpVelNotchInpVal
  FixdToFloat_f32_u16 : FixdToFloat/FixdToFloat_f32_u16  RequirementInfo="{'linktype_rmi_doors' '0000a52e (/E-STEER Core/SubSystem Specifications/Application Functions/SF014A Inertia Compensation)' '#SF014A_92' 'true' 'REQ:  SF014A_92' '' } %GIDa_d4c074de_6c39_4d70_ad9b_f8af722abd74"  Param1=15
  FloatToFixd_u16_f1 : FloatToFixd/FloatToFixd_u16_f32  RequirementInfo="{'linktype_rmi_doors' '0000a52e (/E-STEER Core/SubSystem Specifications/Application Functions/SF014A Inertia Compensation)' '#SF014A_92' 'true' 'REQ:  SF014A_92' '' } %GIDa_70a70d87_38d2_490d_a032_97c9dab3bca1"  Param1=7
  LnrIntrpn_u16_u16VariXu16VariY : LnrIntrpn/LnrIntrpn_u16_u16VariXu16VariY  RequirementInfo="{'linktype_rmi_doors' '0000a52e (/E-STEER Core/SubSystem Specifications/Application Functions/SF014A Inertia Compensation)' '#SF014A_92' 'true' 'REQ:  SF014A_92' '' } %GIDa_f5844dd4_b25e_4a3f_9c1d_81e8adc88314"  XTbl=SysGlbPrmVehSpdBilnrSeln  YTbl=InertiaCmpVelNotchBlndY
      settings: AttributesFormatString=Lnr ( u16VariX , u16VariY )
  NotchFilter : Subsystem
  InertiaCompcompensated : Outport
  wires:
  InertiaComp/1 -> NotchFilter/1(InertiaComp), Blnd_f32/1, Data Store Write3/1
  NotchFilter/1(CompVelOutp) -> Data Store Write2/1, Blnd_f32/2
  FixdToFloat_f32_u16/1 -> Data Store Write1/1, Blnd_f32/3
  LnrIntrpn_u16_u16VariXu16VariY/1 -> FixdToFloat_f32_u16/1
  FloatToFixd_u16_f1/1 -> LnrIntrpn_u16_u16VariXu16VariY/1
  VehSpd/1 -> FloatToFixd_u16_f1/1
  Blnd_f32/1 -> InertiaCompcompensated/1

== system SF014A_InertiaCmpVel/InertiaCmpVel/InertiaCmpVelPer1/InertiaCmpVelCmdDisable ==
  Action Port : ActionPort  ActionType=then
  Constant : Constant  Value=0  OutDataTypeStr=single
      settings: AttributesFormatString=%<OutDataTypeStr>
  CopyRight2 : Subsystem  Description=|  mask(Copyright Information){none=on}
      | Copyright info block.                                               
      |                                                                     
      | Place copyright information at the top of every subsystem in design.
      mask prompts: none "No parameters"
      mask help: Place copyright information at the top of every subsystem in design.
      mask Display:
      | NxtrConf = 'Nexteer Confidential';
      | 
      | sys = bdroot; %handle for the current model ("system")
      | first = get_param(sys,'Created');
      | first = first(end-3:end);  %year is last four digits
      | 
      | last = get_param(sys,'LastModifiedDate');
      | if isempty(last)
      |     last = datestr(now,'yyyy');
      | else
      |     last = last(end-3:end);
      | end
      | 
      | if strcmp(first,last)
      |     fprintf('%s -- Copyright %s Nexteer',NxtrConf,first)
      | else
      |     fprintf('%s -- %s%s- %s Nexteer',NxtrConf,char(169),first,last)
      | end
  InertiaCmpVelCmd : Outport
  wires:
  Constant/1 -> InertiaCmpVelCmd/1

== system SF014A_InertiaCmpVel/InertiaCmpVel/InertiaCmpVelPer1/InertiaCmpVelCmdEnable ==
  InertiaCompcompensated : Inport
  Action Port : ActionPort  ActionType=else
  CopyRight2 : Subsystem  Description=|  mask(Copyright Information){none=on}
      | Copyright info block.                                               
      |                                                                     
      | Place copyright information at the top of every subsystem in design.
      mask prompts: none "No parameters"
      mask help: Place copyright information at the top of every subsystem in design.
      mask Display:
      | NxtrConf = 'Nexteer Confidential';
      | 
      | sys = bdroot; %handle for the current model ("system")
      | first = get_param(sys,'Created');
      | first = first(end-3:end);  %year is last four digits
      | 
      | last = get_param(sys,'LastModifiedDate');
      | if isempty(last)
      |     last = datestr(now,'yyyy');
      | else
      |     last = last(end-3:end);
      | end
      | 
      | if strcmp(first,last)
      |     fprintf('%s -- Copyright %s Nexteer',NxtrConf,first)
      | else
      |     fprintf('%s -- %s%s- %s Nexteer',NxtrConf,char(169),first,last)
      | end
  InertiaCmpVelCmd : Outport
  wires:
  InertiaCompcompensated/1 -> InertiaCmpVelCmd/1

== system SF014A_InertiaCmpVel/InertiaCmpVel/InertiaCmpVelInit1/NotchFilterDisable/CopyRight2 ==

== system SF014A_InertiaCmpVel/InertiaCmpVel/InertiaCmpVelInit1/NotchFilterEnable/CopyRight2 ==

== system SF014A_InertiaCmpVel/InertiaCmpVel/InertiaCmpVelPer1/ADDCoefCalc/CopyRight2 ==

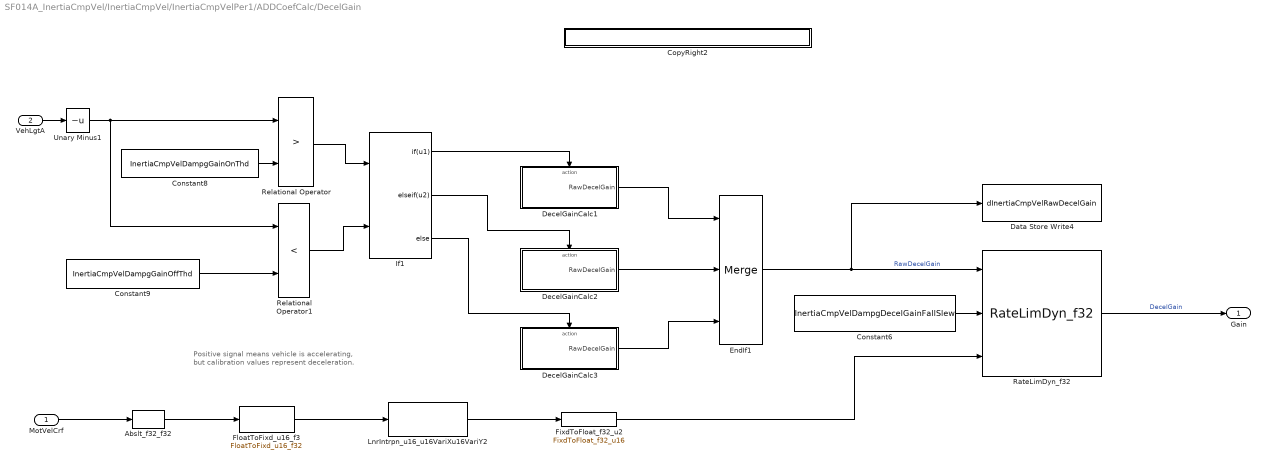
== system SF014A_InertiaCmpVel/InertiaCmpVel/InertiaCmpVelPer1/ADDCoefCalc/DecelGain ==
  note: Positive signal means vehicle is accelerating,
      | but calibration values represent deceleration.
  MotVelCrf : Inport
  VehLgtA : Inport  Port=2
  Abslt_f32_f32 : NxtrAbslt/Abslt_f32_f32  SFunctionSpec=single y1 = Abslt_f32_f32(single u1)
      settings: AttributesFormatString=%<Name>
  Constant6 : Constant  Value=InertiaCmpVelDampgDecelGainFallSlew
  Constant8 : Constant  Value=InertiaCmpVelDampgGainOnThd
  Constant9 : Constant  Value=InertiaCmpVelDampgGainOffThd
  CopyRight2 : Subsystem  Description=|  mask(Copyright Information){none=on}
      | Copyright info block.                                               
      |                                                                     
      | Place copyright information at the top of every subsystem in design.
      mask prompts: none "No parameters"
      mask help: Place copyright information at the top of every subsystem in design.
      mask Display:
      | NxtrConf = 'Nexteer Confidential';
      | 
      | sys = bdroot; %handle for the current model ("system")
      | first = get_param(sys,'Created');
      | first = first(end-3:end);  %year is last four digits
      | 
      | last = get_param(sys,'LastModifiedDate');
      | if isempty(last)
      |     last = datestr(now,'yyyy');
      | else
      |     last = last(end-3:end);
      | end
      | 
      | if strcmp(first,last)
      |     fprintf('%s -- Copyright %s Nexteer',NxtrConf,first)
      | else
      |     fprintf('%s -- %s%s- %s Nexteer',NxtrConf,char(169),first,last)
      | end
  Data Store Write4 : DataStoreWrite  DataStoreName=dInertiaCmpVelRawDecelGain
  DecelGainCalc1 : Subsystem  TreatAsAtomicUnit=on
  DecelGainCalc2 : Subsystem  TreatAsAtomicUnit=on
  DecelGainCalc3 : Subsystem  TreatAsAtomicUnit=on
  EndIf1 : Merge  Inputs=3
  FixdToFloat_f32_u2 : FixdToFloat/FixdToFloat_f32_u16  Param1=3
  FloatToFixd_u16_f3 : FloatToFixd/FloatToFixd_u16_f32  Param1=5
  If1 : If  NumInputs=2  IfExpression=u1  ElseIfExpressions=u2
  LnrIntrpn_u16_u16VariXu16VariY2 : LnrIntrpn/LnrIntrpn_u16_u16VariXu16VariY  XTbl=InertiaCmpVelDampgDecelGainRisngSlewX  YTbl=InertiaCmpVelDampgDecelGainRisngSlewY
      settings: AttributesFormatString=Lnr ( u16VariX , u16VariY )
  RateLimDyn_f32 : NxtrLim/RateLimDyn_f32  StVar=DecelGain  Ts=single(0.002)
      settings: AttributesFormatString=StVar: %<StVar>
  Relational Operator : RelationalOperator  Operator=>  OutDataTypeStr=boolean
  Relational Operator1 : RelationalOperator  Operator=<  OutDataTypeStr=boolean
  Unary Minus1 : UnaryMinus
  Gain : Outport
  wires:
  MotVelCrf/1 -> Abslt_f32_f32/1
  Abslt_f32_f32/1 -> FloatToFixd_u16_f3/1
  DecelGainCalc3/1(RawDecelGain) -> EndIf1/3
  EndIf1/1 -> RateLimDyn_f32/1, Data Store Write4/1  "RawDecelGain"
  RateLimDyn_f32/1 -> Gain/1  "DecelGain"
  Constant6/1 -> RateLimDyn_f32/2
  Relational Operator/1 -> If1/1
  Relational Operator1/1 -> If1/2
  If1/1 -> DecelGainCalc1/Action
  DecelGainCalc1/1(RawDecelGain) -> EndIf1/1
  If1/2 -> DecelGainCalc2/Action
  DecelGainCalc2/1(RawDecelGain) -> EndIf1/2
  If1/3 -> DecelGainCalc3/Action
  LnrIntrpn_u16_u16VariXu16VariY2/1 -> FixdToFloat_f32_u2/1
  FloatToFixd_u16_f3/1 -> LnrIntrpn_u16_u16VariXu16VariY2/1
  FixdToFloat_f32_u2/1 -> RateLimDyn_f32/3
  VehLgtA/1 -> Unary Minus1/1
  Unary Minus1/1 -> Relational Operator/1, Relational Operator1/1
  Constant8/1 -> Relational Operator/2
  Constant9/1 -> Relational Operator1/2

== system SF014A_InertiaCmpVel/InertiaCmpVel/InertiaCmpVelPer1/ADDCoefCalc/DecelGainDisable ==
  Action Port : ActionPort  ActionType=else
  Constant : Constant  OutDataTypeStr=single
      settings: AttributesFormatString=%<OutDataTypeStr>
  CopyRight2 : Subsystem  Description=|  mask(Copyright Information){none=on}
      | Copyright info block.                                               
      |                                                                     
      | Place copyright information at the top of every subsystem in design.
      mask prompts: none "No parameters"
      mask help: Place copyright information at the top of every subsystem in design.
      mask Display:
      | NxtrConf = 'Nexteer Confidential';
      | 
      | sys = bdroot; %handle for the current model ("system")
      | first = get_param(sys,'Created');
      | first = first(end-3:end);  %year is last four digits
      | 
      | last = get_param(sys,'LastModifiedDate');
      | if isempty(last)
      |     last = datestr(now,'yyyy');
      | else
      |     last = last(end-3:end);
      | end
      | 
      | if strcmp(first,last)
      |     fprintf('%s -- Copyright %s Nexteer',NxtrConf,first)
      | else
      |     fprintf('%s -- %s%s- %s Nexteer',NxtrConf,char(169),first,last)
      | end
  DecelGain : Outport
  wires:
  Constant/1 -> DecelGain/1

== system SF014A_InertiaCmpVel/InertiaCmpVel/InertiaCmpVelPer1/ADDCoefCalc/DecelGainEnable ==
  Gain : Inport
  Action Port : ActionPort  ActionType=then
  CopyRight2 : Subsystem  Description=|  mask(Copyright Information){none=on}
      | Copyright info block.                                               
      |                                                                     
      | Place copyright information at the top of every subsystem in design.
      mask prompts: none "No parameters"
      mask help: Place copyright information at the top of every subsystem in design.
      mask Display:
      | NxtrConf = 'Nexteer Confidential';
      | 
      | sys = bdroot; %handle for the current model ("system")
      | first = get_param(sys,'Created');
      | first = first(end-3:end);  %year is last four digits
      | 
      | last = get_param(sys,'LastModifiedDate');
      | if isempty(last)
      |     last = datestr(now,'yyyy');
      | else
      |     last = last(end-3:end);
      | end
      | 
      | if strcmp(first,last)
      |     fprintf('%s -- Copyright %s Nexteer',NxtrConf,first)
      | else
      |     fprintf('%s -- %s%s- %s Nexteer',NxtrConf,char(169),first,last)
      | end
  DecelGain : Outport
  wires:
  Gain/1 -> DecelGain/1

== system SF014A_InertiaCmpVel/InertiaCmpVel/InertiaCmpVelPer1/DriverVelCalc/CopyRight2 ==

== system SF014A_InertiaCmpVel/InertiaCmpVel/InertiaCmpVelPer1/FilterCoefCalc/Coeff_a0 ==
  FilFreqRadPs : Inport
  Constant12 : Constant  Value=2  OutDataTypeStr=single
      settings: AttributesFormatString=%<OutDataTypeStr>
  Constant7 : Constant  Value=ARCHGLBPRM_2MILLISEC_SEC_F32
  CopyRight2 : Subsystem  Description=|  mask(Copyright Information){none=on}
      | Copyright info block.                                               
      |                                                                     
      | Place copyright information at the top of every subsystem in design.
      mask prompts: none "No parameters"
      mask help: Place copyright information at the top of every subsystem in design.
      mask Display:
      | NxtrConf = 'Nexteer Confidential';
      | 
      | sys = bdroot; %handle for the current model ("system")
      | first = get_param(sys,'Created');
      | first = first(end-3:end);  %year is last four digits
      | 
      | last = get_param(sys,'LastModifiedDate');
      | if isempty(last)
      |     last = datestr(now,'yyyy');
      | else
      |     last = last(end-3:end);
      | end
      | 
      | if strcmp(first,last)
      |     fprintf('%s -- Copyright %s Nexteer',NxtrConf,first)
      | else
      |     fprintf('%s -- %s%s- %s Nexteer',NxtrConf,char(169),first,last)
      | end
  Math Function5 : Math  Operator=square  SaturateOnIntegerOverflow=on
  Product26 : Product  Inputs=**  RndMeth=Zero  OutDataTypeStr=Inherit: Same as first input
  Sum15 : Sum  Inputs=-+  OutDataTypeStr=Inherit: Same as first input
  a0 : Outport
  wires:
  FilFreqRadPs/1 -> Product26/1
  Constant7/1 -> Product26/2
  Sum15/1 -> Math Function5/1
  Math Function5/1 -> a0/1  "a0"
  Product26/1 -> Sum15/2
  Constant12/1 -> Sum15/1

== system SF014A_InertiaCmpVel/InertiaCmpVel/InertiaCmpVelPer1/FilterCoefCalc/Coeff_a1 ==
  FilFreqRadPs : Inport
  Constant15 : Constant  Value=4  OutDataTypeStr=single
      settings: AttributesFormatString=%<OutDataTypeStr>
  Constant18 : Constant  Value=2  OutDataTypeStr=single
      settings: AttributesFormatString=%<OutDataTypeStr>
  Constant8 : Constant  Value=ARCHGLBPRM_2MILLISEC_SEC_F32
  CopyRight2 : Subsystem  Description=|  mask(Copyright Information){none=on}
      | Copyright info block.                                               
      |                                                                     
      | Place copyright information at the top of every subsystem in design.
      mask prompts: none "No parameters"
      mask help: Place copyright information at the top of every subsystem in design.
      mask Display:
      | NxtrConf = 'Nexteer Confidential';
      | 
      | sys = bdroot; %handle for the current model ("system")
      | first = get_param(sys,'Created');
      | first = first(end-3:end);  %year is last four digits
      | 
      | last = get_param(sys,'LastModifiedDate');
      | if isempty(last)
      |     last = datestr(now,'yyyy');
      | else
      |     last = last(end-3:end);
      | end
      | 
      | if strcmp(first,last)
      |     fprintf('%s -- Copyright %s Nexteer',NxtrConf,first)
      | else
      |     fprintf('%s -- %s%s- %s Nexteer',NxtrConf,char(169),first,last)
      | end
  Math Function6 : Math  Operator=square  SaturateOnIntegerOverflow=on
  Product27 : Product  Inputs=**  RndMeth=Zero  OutDataTypeStr=Inherit: Same as first input
  Product9 : Product  Inputs=**  RndMeth=Zero  OutDataTypeStr=Inherit: Same as first input
  Sum16 : Sum  Inputs=-+  OutDataTypeStr=Inherit: Same as first input
  a1 : Outport
  wires:
  FilFreqRadPs/1 -> Product27/1
  Constant8/1 -> Product27/2
  Constant15/1 -> Sum16/1
  Product27/1 -> Math Function6/1
  Sum16/1 -> Product9/1
  Math Function6/1 -> Sum16/2
  Product9/1 -> a1/1  "a1"
  Constant18/1 -> Product9/2
